simulink model "HAC_swingUp_controller"  (R2022b)
settings: Solver=VariableStepAuto  StartTime=0.0  StopTime=10.0  RelTol=1e-3
undefined symbols (not defined in the file): E_up, eta, g, I, interp_x, interp_y, k_cw, k_em, k_su, k_vw, L, m, q_d_kt, q_kt, u_kt, uMax, x1_max, x2_max, x_d_kt, x_kt
settings Model: Creator=doann  LastModifiedBy=doann
settings OptimizationCC: DefaultParameterBehavior=Inlined  UseDivisionForNetSlopeComputation=on  GainParamInheritBuiltInType=on  UseFloatMulNetSlope=on  InlineInvariantSignals=on  PassReuseOutputArgsAs=Individual arguments  ZeroExternalMemoryAtStartup=off  ZeroInternalMemoryAtStartup=off  NoFixptDivByZeroProtection=on  EfficientFloat2IntCast=on  LifeSpan=1  OptimizeBlockOrder=speed  DifferentSizesBufferReuse=on  EfficientTunableParamExpr=on
settings DebuggingCC: ParameterTunabilityLossMsg=error
settings HardwareCC: ProdBitPerPointer=32  ProdBitPerSizeT=32  ProdBitPerPtrDiffT=32  ProdLargestAtomicInteger=Long  ProdLargestAtomicFloat=Double  ProdWordSize=32  ProdLongLongMode=on  ProdHWDeviceType=ARM Compatible->ARM Cortex-M
settings SFSimCC: MATLABDynamicMemAlloc=off
settings RTWCC: Description=Embedded Coder  SystemTargetFile=ert.tlc  TemplateMakefile=ert_default_tmf  TargetLang=C++
settings CodeAppCC: ForceParamTrailComments=on  IgnoreCustomStorageClasses=off  OperatorAnnotations=on  SimulinkDataObjDesc=on  SFDataObjDesc=on  CustomSymbolStrGlobalVar=rt$N$M  CustomSymbolStrType=$N$M  CustomSymbolStrFcn=$N$M$F  CustomSymbolStrMacro=$N$M  InsertBlockDesc=on
settings ERTTargetCC: TargetLangStandard=C++11 (ISO)  GenerateSampleERTMain=on  IncludeMdlTerminateFcn=off  CombineSignalStateStructs=on  SuppressErrorStatus=on  SupportAbsoluteTime=off  CodeInterfacePackaging=C++ class  SupportComplex=off  InlinedParameterPlacement=NonHierarchical  RootIOFormat=Structure reference  ERTCustomFileTemplate=example_file_process.tlc  ERTFilePackagingFormat=CompactWithDataFile

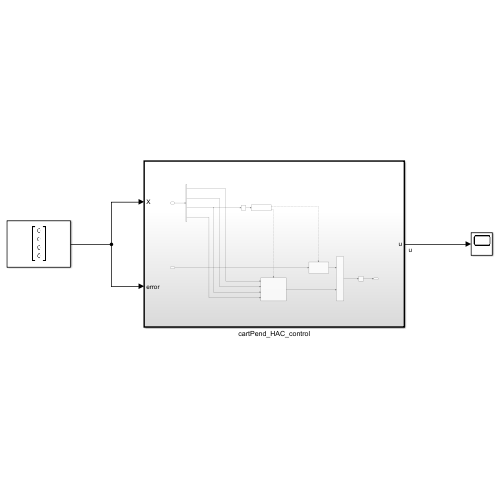
[thumbnail: Simulink's stored preview of the top-level diagram]
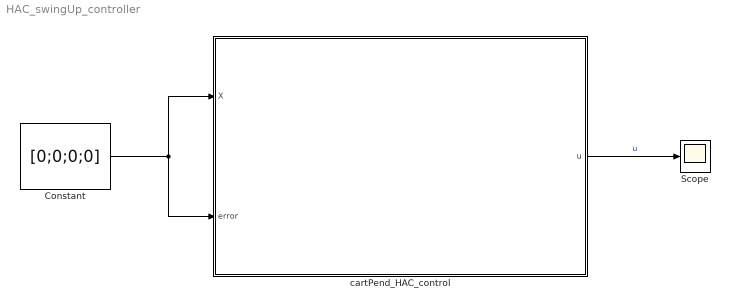
== system HAC_swingUp_controller ==
  Constant : Constant  Value=[0;0;0;0]  VectorParams1D=off
  Scope : Scope
  cartPend_HAC_control : Subsystem  TreatAsAtomicUnit=on  SystemSampleTime=0.001
  wires:
  Constant/1 -> cartPend_HAC_control/1(X), cartPend_HAC_control/2(error)
  cartPend_HAC_control/1(u) -> Scope/1  "u"

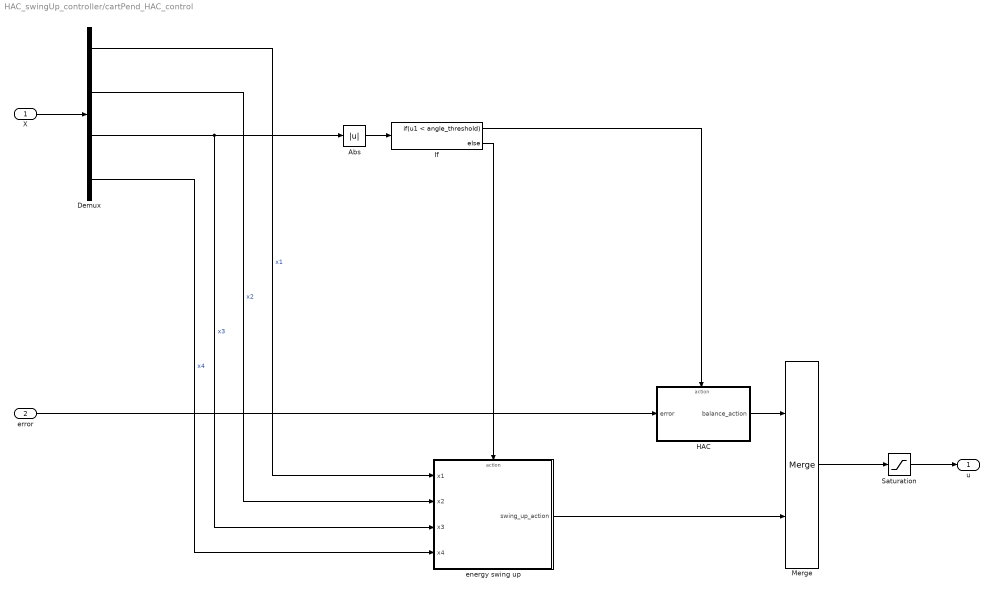
== system HAC_swingUp_controller/cartPend_HAC_control ==
  X : Inport
  error : Inport  Port=2
  Abs : Abs  SaturateOnIntegerOverflow=off
  Demux : Demux
  HAC : Subsystem  TreatAsAtomicUnit=on
  If : If  IfExpression=u1 < angle_threshold
  Merge : Merge
  Saturation : Saturate  UpperLimit=uMax  LowerLimit=-uMax
  energy swing up : Subsystem  TreatAsAtomicUnit=on
  u : Outport
  wires:
  X/1 -> Demux/1
  Demux/3 -> Abs/1, energy swing up/3(x3)  "x3"
  Demux/4 -> energy swing up/4(x4)  "x4"
  Abs/1 -> If/1
  If/1 -> HAC/Action
  If/2 -> energy swing up/Action
  HAC/1(balance_action) -> Merge/1
  energy swing up/1(swing_up_action) -> Merge/2
  error/1 -> HAC/1(error)
  Demux/2 -> energy swing up/2(x2)  "x2"
  Demux/1 -> energy swing up/1(x1)  "x1"
  Merge/1 -> Saturation/1
  Saturation/1 -> u/1

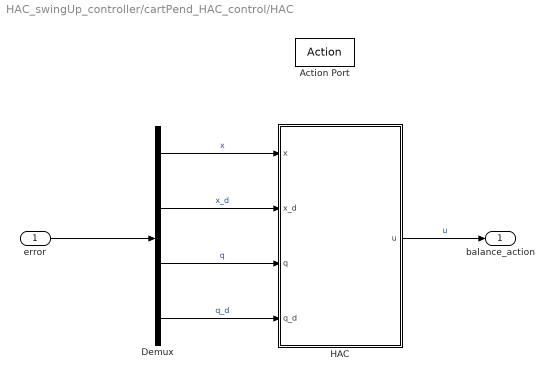
== system HAC_swingUp_controller/cartPend_HAC_control/HAC ==
  error : Inport
  Action Port : ActionPort  ActionPortLabel=if(u1 < angle_threshold)
  Demux : Demux
  HAC : Subsystem
  balance_action : Outport
  wires:
  HAC/1(u) -> balance_action/1  "u"
  error/1 -> Demux/1
  Demux/4 -> HAC/4(q_d)  "q_d"
  Demux/3 -> HAC/3(q)  "q"
  Demux/2 -> HAC/2(x_d)  "x_d"
  Demux/1 -> HAC/1(x)  "x"

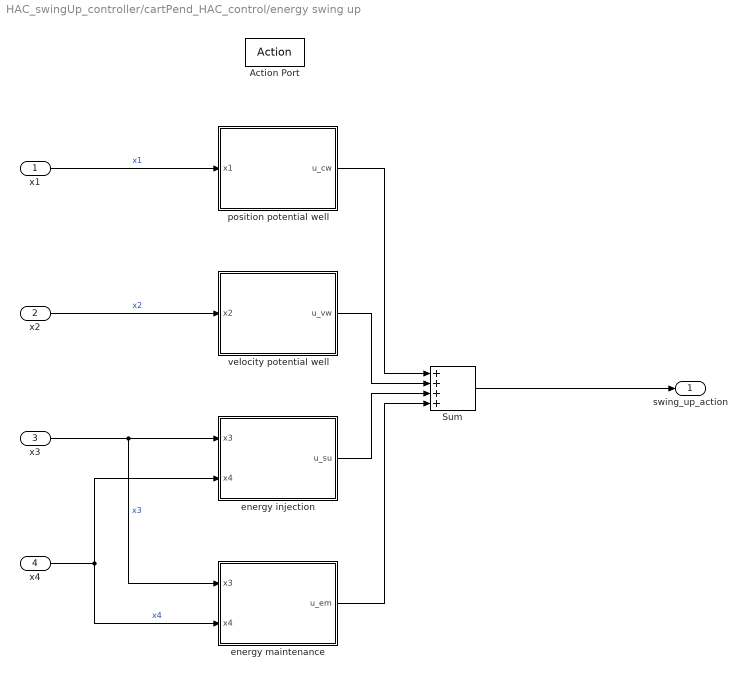
== system HAC_swingUp_controller/cartPend_HAC_control/energy swing up ==
  x1 : Inport
  x2 : Inport  Port=2
  x3 : Inport  Port=3
  x4 : Inport  Port=4
  Action Port : ActionPort  ActionPortLabel=else
  Sum : Sum  Inputs=++++
  energy injection : Subsystem
  energy maintenance : Subsystem
  position potential well : Subsystem
  velocity potential well : Subsystem
  swing_up_action : Outport
  wires:
  energy injection/1(u_su) -> Sum/3
  x2/1 -> velocity potential well/1(x2)  "x2"
  velocity potential well/1(u_vw) -> Sum/2
  Sum/1 -> swing_up_action/1
  energy maintenance/1(u_em) -> Sum/4
  x3/1 -> energy maintenance/1(x3), energy injection/1(x3)  "x3"
  x1/1 -> position potential well/1(x1)  "x1"
  x4/1 -> energy injection/2(x4), energy maintenance/2(x4)  "x4"
  position potential well/1(u_cw) -> Sum/1

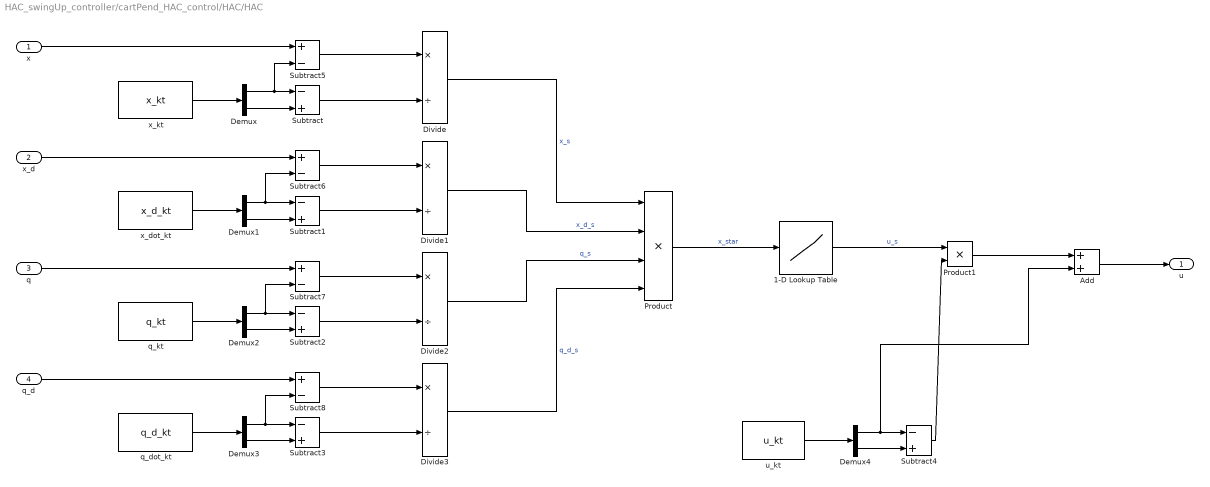
== system HAC_swingUp_controller/cartPend_HAC_control/HAC/HAC ==
  x : Inport
  x_d : Inport  Port=2
  q : Inport  Port=3
  q_d : Inport  Port=4
  1-D Lookup Table : Lookup_n-D  NumberOfTableDimensions=1  BreakpointsForDimension1=interp_x  Table=interp_y  InterpMethod=Cubic spline  InternalRulePriority=Speed  RndMeth=Simplest
  Add : Sum
  Demux{,1..4} (5 alike) : Demux  Outputs=2
  Divide{,1..3} (4 alike) : Product  Inputs=*/
  Product : Product  Inputs=4
  Product1 : Product
  Subtract{,1..4} (5 alike) : Sum  Inputs=-+
  Subtract{5..8} (4 alike) : Sum  Inputs=+-
  q_dot_kt : Constant  Value=q_d_kt  VectorParams1D=off
  q_kt : Constant  Value=q_kt  VectorParams1D=off
  u_kt : Constant  Value=u_kt  VectorParams1D=off
  x_dot_kt : Constant  Value=x_d_kt  VectorParams1D=off
  x_kt : Constant  Value=x_kt  VectorParams1D=off
  u : Outport
  wires:
  Subtract2/1 -> Divide2/2
  Subtract4/1 -> Product1/2
  q_kt/1 -> Demux2/1
  q_dot_kt/1 -> Demux3/1
  Demux2/2 -> Subtract2/2
  Demux4/2 -> Subtract4/2
  Demux4/1 -> Add/2, Subtract4/1
  q_d/1 -> Subtract8/1
  Divide3/1 -> Product/4  "q_d_s"
  Add/1 -> u/1
  q/1 -> Subtract7/1
  Divide/1 -> Product/1  "x_s"
  x/1 -> Subtract5/1
  Subtract1/1 -> Divide1/2
  u_kt/1 -> Demux4/1
  Demux/2 -> Subtract/2
  Demux1/2 -> Subtract1/2
  Subtract3/1 -> Divide3/2
  Demux/1 -> Subtract/1, Subtract5/2
  Subtract5/1 -> Divide/1
  Subtract/1 -> Divide/2
  x_kt/1 -> Demux/1
  x_d/1 -> Subtract6/1
  Demux3/1 -> Subtract3/1, Subtract8/2
  Divide2/1 -> Product/3  "q_s"
  Demux1/1 -> Subtract1/1, Subtract6/2
  1-D Lookup Table/1 -> Product1/1  "u_s"
  Subtract6/1 -> Divide1/1
  Divide1/1 -> Product/2  "x_d_s"
  Subtract8/1 -> Divide3/1
  x_dot_kt/1 -> Demux1/1
  Demux3/2 -> Subtract3/2
  Product/1 -> 1-D Lookup Table/1  "x_star"
  Subtract7/1 -> Divide2/1
  Demux2/1 -> Subtract2/1, Subtract7/2
  Product1/1 -> Add/1

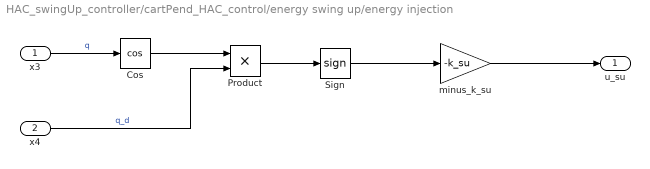
== system HAC_swingUp_controller/cartPend_HAC_control/energy swing up/energy injection ==
  x3 : Inport
  x4 : Inport  Port=2
  Cos : Trigonometry  Operator=cos
  Product : Product
  Sign : Signum
  minus_k_su : Gain  Gain=-k_su
  u_su : Outport
  wires:
  x3/1 -> Cos/1  "q"
  x4/1 -> Product/2  "q_d"
  Sign/1 -> minus_k_su/1
  minus_k_su/1 -> u_su/1
  Cos/1 -> Product/1
  Product/1 -> Sign/1

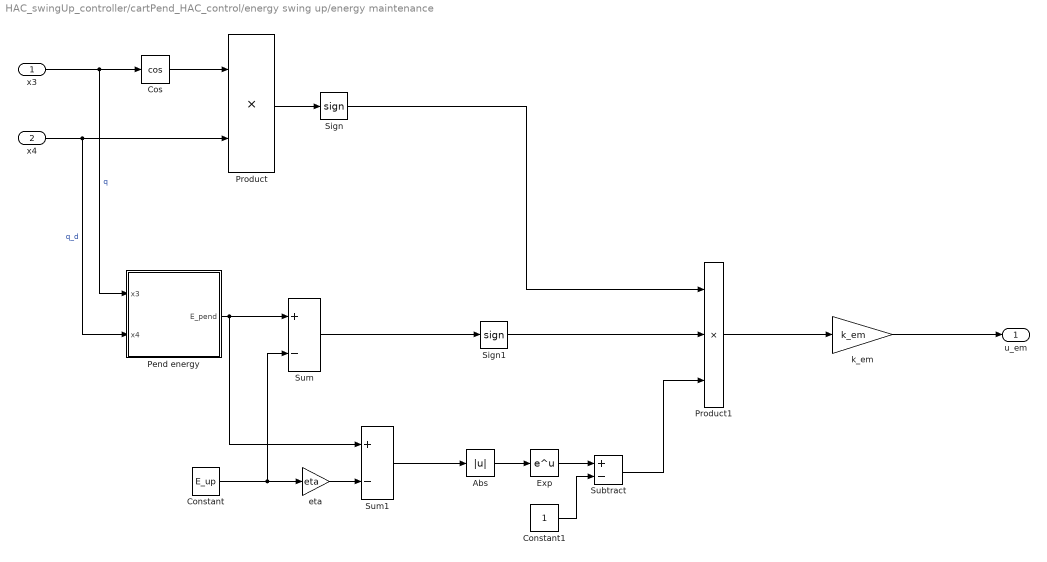
== system HAC_swingUp_controller/cartPend_HAC_control/energy swing up/energy maintenance ==
  x3 : Inport
  x4 : Inport  Port=2
  Abs : Abs  SaturateOnIntegerOverflow=off
  Constant : Constant  Value=E_up
  Constant1 : Constant
  Cos : Trigonometry  Operator=cos
  Exp : Math
  Pend energy : Subsystem
  Product : Product
  Product1 : Product  Inputs=3
  Sign : Signum
  Sign1 : Signum
  Subtract : Sum  Inputs=+-
  Sum : Sum  Inputs=+-
  Sum1 : Sum  Inputs=+-
  eta : Gain  Gain=eta
  k_em : Gain  Gain=k_em
  u_em : Outport
  wires:
  x3/1 -> Pend energy/1(x3), Cos/1  "q"
  Cos/1 -> Product/1
  x4/1 -> Pend energy/2(x4), Product/2  "q_d"
  Product/1 -> Sign/1
  Pend energy/1(E_pend) -> Sum/1, Sum1/1
  Constant/1 -> Sum/2, eta/1
  Sum/1 -> Sign1/1
  eta/1 -> Sum1/2
  Sum1/1 -> Abs/1
  Abs/1 -> Exp/1
  Exp/1 -> Subtract/1
  Constant1/1 -> Subtract/2
  Sign1/1 -> Product1/2
  Sign/1 -> Product1/1
  Subtract/1 -> Product1/3
  Product1/1 -> k_em/1
  k_em/1 -> u_em/1

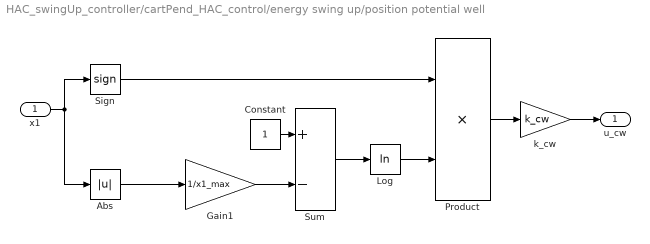
== system HAC_swingUp_controller/cartPend_HAC_control/energy swing up/position potential well ==
  x1 : Inport
  Abs : Abs  SaturateOnIntegerOverflow=off
  Constant : Constant
  Gain1 : Gain  Gain=1/x1_max
  Log : Math  Operator=log
  Product : Product
  Sign : Signum
  Sum : Sum  Inputs=+-
  k_cw : Gain  Gain=k_cw
  u_cw : Outport
  wires:
  x1/1 -> Abs/1, Sign/1
  Abs/1 -> Gain1/1
  Gain1/1 -> Sum/2
  Constant/1 -> Sum/1
  Sum/1 -> Log/1
  k_cw/1 -> u_cw/1
  Product/1 -> k_cw/1
  Log/1 -> Product/2
  Sign/1 -> Product/1

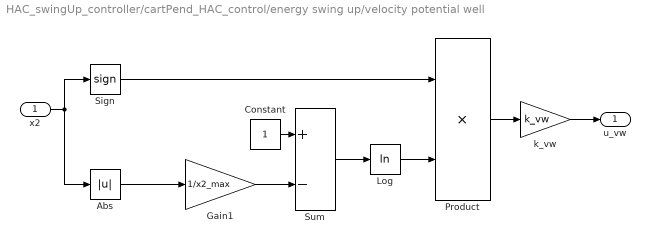
== system HAC_swingUp_controller/cartPend_HAC_control/energy swing up/velocity potential well ==
  x2 : Inport
  Abs : Abs  SaturateOnIntegerOverflow=off
  Constant : Constant
  Gain1 : Gain  Gain=1/x2_max
  Log : Math  Operator=log
  Product : Product
  Sign : Signum
  Sum : Sum  Inputs=+-
  k_vw : Gain  Gain=k_vw
  u_vw : Outport
  wires:
  Sign/1 -> Product/1
  Log/1 -> Product/2
  Product/1 -> k_vw/1
  k_vw/1 -> u_vw/1
  Sum/1 -> Log/1
  Constant/1 -> Sum/1
  Gain1/1 -> Sum/2
  Abs/1 -> Gain1/1
  x2/1 -> Sign/1, Abs/1

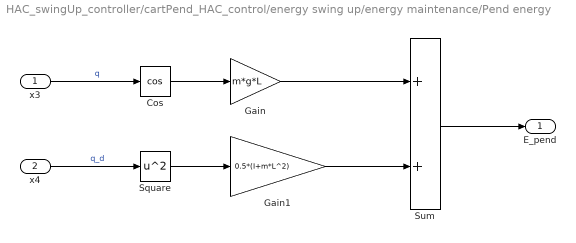
== system HAC_swingUp_controller/cartPend_HAC_control/energy swing up/energy maintenance/Pend energy ==
  x3 : Inport
  x4 : Inport  Port=2
  Cos : Trigonometry  Operator=cos
  Gain : Gain  Gain=m*g*L
  Gain1 : Gain  Gain=0.5*(I+m*L^2)
  Square : Math  Operator=square
  Sum : Sum
  E_pend : Outport
  wires:
  x3/1 -> Cos/1  "q"
  x4/1 -> Square/1  "q_d"
  Cos/1 -> Gain/1
  Square/1 -> Gain1/1
  Gain/1 -> Sum/1
  Gain1/1 -> Sum/2
  Sum/1 -> E_pend/1
